simulink model "MovimientoRotacional"  (R2024a)
settings: Solver=VariableStepAuto  StartTime=0.0  StopTime=10.0  RelTol=1e-3

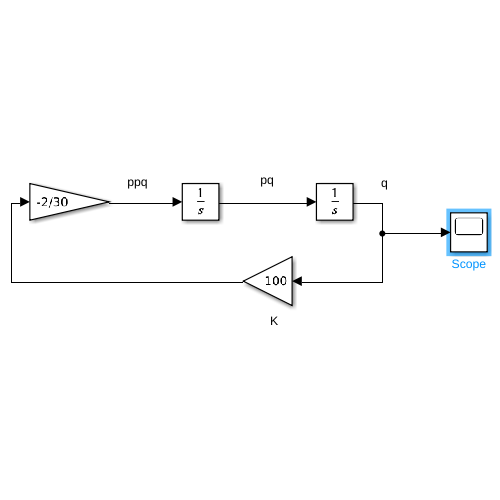
[thumbnail: Simulink's stored preview of the top-level diagram]
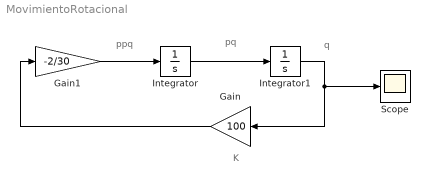
== system MovimientoRotacional ==
  note: pq
  note: ppq
  note: q
  note: K
  Gain : Gain  Gain=100
  Gain1 : Gain  Gain=-2/30
  Integrator : Integrator  InitialCondition=2
  Integrator1 : Integrator
  Scope : Scope
  wires:
  Integrator/1 -> Integrator1/1
  Integrator1/1 -> Scope/1, Gain/1
  Gain1/1 -> Integrator/1
  Gain/1 -> Gain1/1
